simulink model "Linear_wObserver"  (R2022a)
settings: Solver=VariableStepAuto  StartTime=0.16733  StopTime=3000.0185  RelTol=1e-3
undefined symbols (not defined in the file): A_HD, A_platform, B_HD, B_platform, C_HD, C_out, C_platform, HD_FOP, L_platform
settings Model: Creator=ianam  LastModifiedBy=ianam
settings DataIOCC: InitialState=IC  LoadInitialState=on
settings DebuggingCC: UnderSpecifiedDataTypeMsg=error  UnderSpecifiedDimensionMsg=error

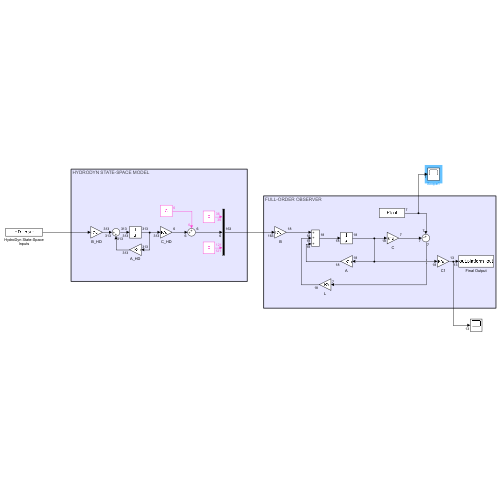
[thumbnail: Simulink's stored preview of the top-level diagram]
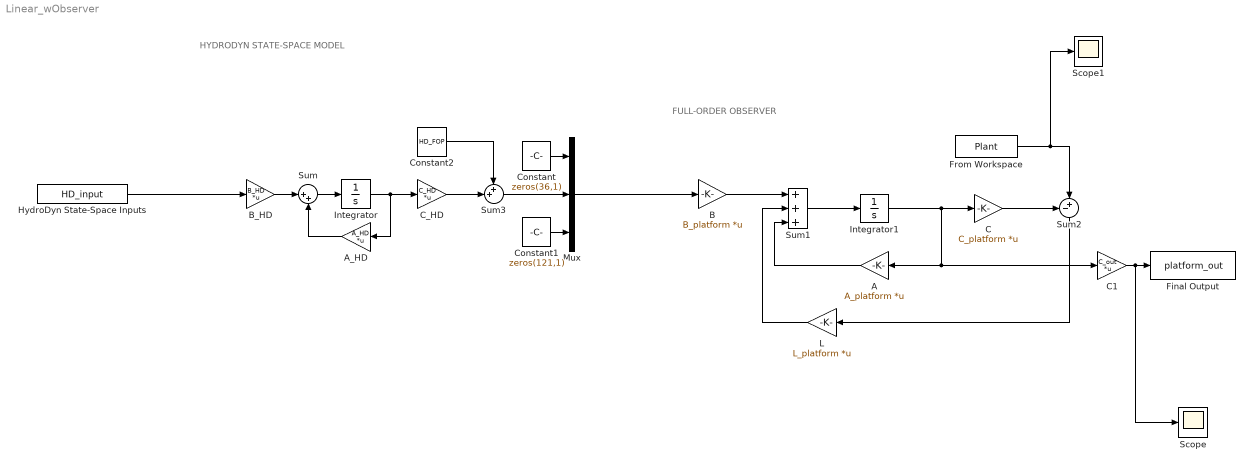
== system Linear_wObserver ==
  note: HYDRODYN STATE-SPACE MODEL
  note: FULL-ORDER OBSERVER
  A : Gain  Gain=A_platform  Multiplication=Matrix(K*u)
  A_HD : Gain  Gain=A_HD  Multiplication=Matrix(K*u)
  B : Gain  Gain=B_platform  Multiplication=Matrix(K*u)
  B_HD : Gain  Gain=B_HD  Multiplication=Matrix(K*u)
  C : Gain  Gain=C_platform  Multiplication=Matrix(K*u)
  C1 : Gain  Gain=C_out  Multiplication=Matrix(K*u)
  C_HD : Gain  Gain=C_HD  Multiplication=Matrix(K*u)
  Constant : Constant  Value=zeros(36,1)
  Constant1 : Constant  Value=zeros(121,1)
  Constant2 : Constant  Value=HD_FOP
  Final Output : ToWorkspace  VariableName=platform_out  SaveFormat=Timeseries  SampleTime=-1
  From Workspace : FromWorkspace  VariableName=Plant
  HydroDyn State-Space Inputs : FromWorkspace  VariableName=HD_input
  Integrator : Integrator
  Integrator1 : Integrator
  L : Gain  Gain=L_platform  Multiplication=Matrix(K*u)
  Mux : Mux  Inputs=3
  Scope : Scope
  Scope1 : Scope
  Sum : Sum  Inputs=|++
  Sum1 : Sum  Inputs=+++
  Sum2 : Sum  Inputs=-+|
  Sum3 : Sum  Inputs=++|
  wires:
  Sum/1 -> Integrator/1
  Integrator/1 -> C_HD/1, A_HD/1
  A_HD/1 -> Sum/2
  B_HD/1 -> Sum/1
  Sum1/1 -> Integrator1/1
  HydroDyn State-Space Inputs/1 -> B_HD/1
  B/1 -> Sum1/1
  Constant/1 -> Mux/1
  Constant1/1 -> Mux/3
  Integrator1/1 -> C1/1, A/1, C/1
  Mux/1 -> B/1
  C_HD/1 -> Sum3/2
  Sum3/1 -> Mux/2
  Constant2/1 -> Sum3/1
  C/1 -> Sum2/1
  Sum2/1 -> L/1
  A/1 -> Sum1/3
  L/1 -> Sum1/2
  From Workspace/1 -> Scope1/1, Sum2/2
  C1/1 -> Scope/1, Final Output/1
